simulink model "VCMGCM1962020b_v2"  (R2020b)
settings: Solver=FixedStepDiscrete  StartTime=0.0  StopTime=10.0  FixedStep=0.005  RelTol=1e-3  EnableMultiTasking=on
PreLoadFcn:
  | try, model_open; catch, disp('Error occurred while executing model pre-load callback: model_open.m'); disp('Please assure that the MATLAB working directory is set to the model directory before opening.'); end
InitFcn:
  | try, model_open; catch, end
undefined symbols (not defined in the file): Bridge, GCM, H, raptor_get_param_eval, raptor_get_safe_string, raptor_xcp_function
libraries: Blocks_lib x1165, Raptor_lib x665, simulink x62, VCM_lib x5
(part 6 of 23)

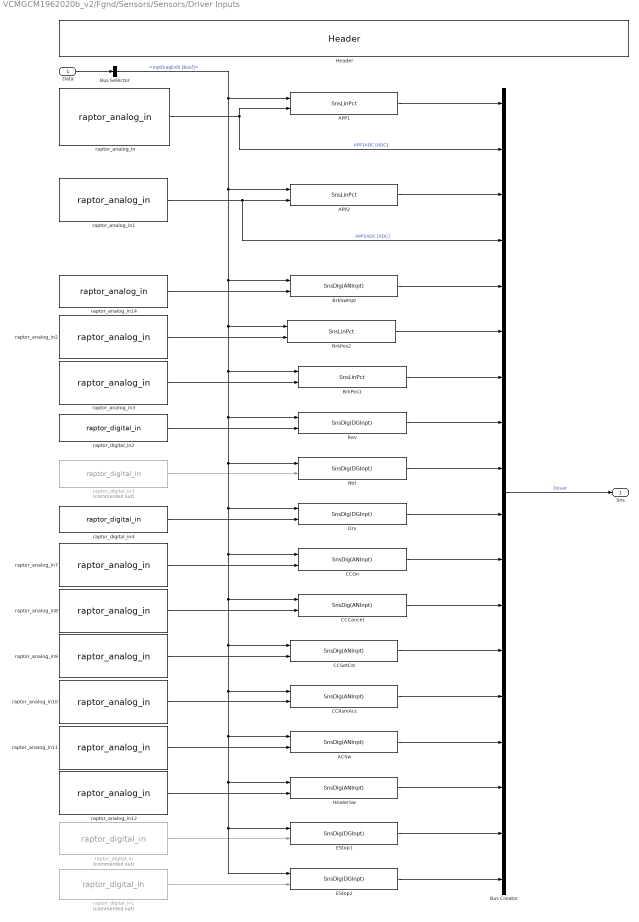
== system VCMGCM1962020b_v2/Fgnd/Sensors/Sensors/Driver Inputs ==
  Data : Inport
  ACSw : Blocks_lib/SnsDig(ANInpt)  nam='ACSw'  group='Sensors | Driver Input'  samptime=samptime
  APP1 : Blocks_lib/SnsLinPct  input=Analog  nam='APP1'  group='Sensors | Driver Input'  samptime=samptime
  APP2 : Blocks_lib/SnsLinPct  input=Analog  nam='APP2'  group='Sensors | Driver Input'  samptime=samptime
  BrkPos1 : Blocks_lib/SnsLinPct  input=Analog  nam='BrkPos1'  group='Sensors | Driver Input'  samptime=samptime
  BrkPos2 : Blocks_lib/SnsLinPct  input=Analog  nam='BrkPos2'  group='Sensors | Driver Input'  samptime=samptime
  BrkSwInpt : Blocks_lib/SnsDig(ANInpt)  nam='BrkSwInpt'  group='Sensors | Driver Input'  samptime=samptime
  Bus Creator : BusCreator  Inputs=18
  Bus Selector : BusSelector  OutputSignals=Control.Mode.StartStop.InptDiagEnbl [Bool]
  CCCancel : Blocks_lib/SnsDig(ANInpt)  nam='CCCancel'  group='Sensors | Driver Input'  samptime=samptime
  CCOn : Blocks_lib/SnsDig(ANInpt)  nam='CCOn'  group='Sensors | Driver Input'  samptime=samptime
  CCRsmAcc : Blocks_lib/SnsDig(ANInpt)  nam='CCRsmAcc'  group='Sensors | Driver Input'  samptime=samptime
  CCSetCst : Blocks_lib/SnsDig(ANInpt)  nam='CCSetCst'  group='Sensors | Driver Input'  samptime=samptime
  Drv : Blocks_lib/SnsDig(DGInpt)  nam='Drv'  group='Sensors | Driver Input'  samptime=samptime
  EStop1 : Blocks_lib/SnsDig(DGInpt)  nam='EStop1'  group='Sensors | Driver Input'  samptime=samptime
  EStop2 : Blocks_lib/SnsDig(DGInpt)  nam='EStop2'  group='Sensors | Driver Input'  samptime=samptime
  Header : Blocks_lib/Header  width=Portrait  addtext=''
  HeaterSw : Blocks_lib/SnsDig(ANInpt)  nam='HeaterSw'  group='Sensors | Driver Input'  samptime=samptime
  Ntrl : Blocks_lib/SnsDig(DGInpt)  nam='Ntrl'  group='Sensors | Driver Input'  samptime=samptime
  Rev : Blocks_lib/SnsDig(DGInpt)  nam='Rev'  group='Sensors | Driver Input'  samptime=samptime
  raptor_analog_in : Raptor_lib/Input & Output/raptor_analog_in  resourceValues=INPUT2|INPUT3|INPUT4|INPUT5|INPUT6|INPUT7|INPUT8|INPUT9|INPUT10|INPUT11|INPUT12|INPUT13|INPUT14|INPUT15|INPUT16|INPUT17|INPUT18|INPUT19|INPUT20|INPUT21|INPUT22|INPUT23|INPUT24|INPUT25|INPUT26|INPUT27|INPUT28|INPUT29|INPUT30|INPUT31|INPUT32|(None)  resource=INPUT30  pullUDValues=215k PD  pullUD=215k PD  rangeValues=0 - 5 V  range=0 - 5 V  filterrateValues=[]  filterrate='RAPTOR MASK DEFAULT'  resolutionValues=[]  resolution=[]
      settings: SourceProductName=Raptor
  raptor_analog_in1 : Raptor_lib/Input & Output/raptor_analog_in  resourceValues=INPUT2|INPUT3|INPUT4|INPUT5|INPUT6|INPUT7|INPUT8|INPUT9|INPUT10|INPUT11|INPUT12|INPUT13|INPUT14|INPUT15|INPUT16|INPUT17|INPUT18|INPUT19|INPUT20|INPUT21|INPUT22|INPUT23|INPUT24|INPUT25|INPUT26|INPUT27|INPUT28|INPUT29|INPUT30|INPUT31|INPUT32|(None)  resource=INPUT29  pullUDValues=215k PD  pullUD=215k PD  rangeValues=0 - 5 V  range=0 - 5 V  filterrateValues=[]  filterrate='RAPTOR MASK DEFAULT'  resolutionValues=[]  resolution=[]
      settings: SourceProductName=Raptor
  raptor_analog_in{7..10} (4 alike) : Raptor_lib/Input & Output/raptor_analog_in  resourceValues=INPUT2|INPUT3|INPUT4|INPUT5|INPUT6|INPUT7|INPUT8|INPUT9|INPUT10|INPUT11|INPUT12|INPUT13|INPUT14|INPUT15|INPUT16|INPUT17|INPUT18|INPUT19|INPUT20|INPUT21|INPUT22|INPUT23|INPUT24|INPUT25|INPUT26|INPUT27|INPUT28|INPUT29|INPUT30|INPUT31|INPUT32|(None)  resource=(None)  pullUDValues=(None)  pullUD=(None)  rangeValues=(None)  range=(None)  filterrateValues=[]  filterrate='RAPTOR MASK DEFAULT'  resolutionValues=[]  resolution=[]
      settings: SourceProductName=Raptor
  raptor_analog_in11 : Raptor_lib/Input & Output/raptor_analog_in  resourceValues=INPUT2|INPUT3|INPUT4|INPUT5|INPUT6|INPUT7|INPUT8|INPUT9|INPUT10|INPUT11|INPUT12|INPUT13|INPUT14|INPUT15|INPUT16|INPUT17|INPUT18|INPUT19|INPUT20|INPUT21|INPUT22|INPUT23|INPUT24|INPUT25|INPUT26|INPUT27|INPUT28|INPUT29|INPUT30|INPUT31|INPUT32|(None)  resource=INPUT8  pullUDValues=4.64k PU  pullUD=4.64k PU  rangeValues=0 - 5 V  range=0 - 5 V  filterrateValues=[]  filterrate='RAPTOR MASK DEFAULT'  resolutionValues=[]  resolution=[]
      settings: SourceProductName=Raptor
  raptor_analog_in12 : Raptor_lib/Input & Output/raptor_analog_in  resourceValues=INPUT2|INPUT3|INPUT4|INPUT5|INPUT6|INPUT7|INPUT8|INPUT9|INPUT10|INPUT11|INPUT12|INPUT13|INPUT14|INPUT15|INPUT16|INPUT17|INPUT18|INPUT19|INPUT20|INPUT21|INPUT22|INPUT23|INPUT24|INPUT25|INPUT26|INPUT27|INPUT28|INPUT29|INPUT30|INPUT31|INPUT32|(None)  resource=INPUT16  pullUDValues=4.64k PU  pullUD=4.64k PU  rangeValues=0 - 5 V  range=0 - 5 V  filterrateValues=[]  filterrate='RAPTOR MASK DEFAULT'  resolutionValues=[]  resolution=[]
      settings: SourceProductName=Raptor
  raptor_analog_in14 : Raptor_lib/Input & Output/raptor_analog_in  resourceValues=INPUT2|INPUT3|INPUT4|INPUT5|INPUT6|INPUT7|INPUT8|INPUT9|INPUT10|INPUT11|INPUT12|INPUT13|INPUT14|INPUT15|INPUT16|INPUT17|INPUT18|INPUT19|INPUT20|INPUT21|INPUT22|INPUT23|INPUT24|INPUT25|INPUT26|INPUT27|INPUT28|INPUT29|INPUT30|INPUT31|INPUT32|(None)  resource=INPUT17  pullUDValues=422k PD  pullUD=422k PD  rangeValues=0 - 5 V  range=0 - 5 V  filterrateValues=[]  filterrate='RAPTOR MASK DEFAULT'  resolutionValues=[]  resolution=[]
      settings: SourceProductName=Raptor
  raptor_analog_in2 : Raptor_lib/Input & Output/raptor_analog_in  resourceValues=INPUT2|INPUT3|INPUT4|INPUT5|INPUT6|INPUT7|INPUT8|INPUT9|INPUT10|INPUT11|INPUT12|INPUT13|INPUT14|INPUT15|INPUT16|INPUT17|INPUT18|INPUT19|INPUT20|INPUT21|INPUT22|INPUT23|INPUT24|INPUT25|INPUT26|INPUT27|INPUT28|INPUT29|INPUT30|INPUT31|INPUT32|(None)  resource=INPUT24  pullUDValues=56.7k PD  pullUD=56.7k PD  rangeValues=0 - 5 V  range=0 - 5 V  filterrateValues=[]  filterrate='RAPTOR MASK DEFAULT'  resolutionValues=[]  resolution=[]
      settings: SourceProductName=Raptor
  raptor_analog_in3 : Raptor_lib/Input & Output/raptor_analog_in  resourceValues=INPUT2|INPUT3|INPUT4|INPUT5|INPUT6|INPUT7|INPUT8|INPUT9|INPUT10|INPUT11|INPUT12|INPUT13|INPUT14|INPUT15|INPUT16|INPUT17|INPUT18|INPUT19|INPUT20|INPUT21|INPUT22|INPUT23|INPUT24|INPUT25|INPUT26|INPUT27|INPUT28|INPUT29|INPUT30|INPUT31|INPUT32|(None)  resource=INPUT23  pullUDValues=56.7k PD  pullUD=56.7k PD  rangeValues=0 - 5 V  range=0 - 5 V  filterrateValues=[]  filterrate='RAPTOR MASK DEFAULT'  resolutionValues=[]  resolution=[]
      settings: SourceProductName=Raptor
  raptor_digital_in : Raptor_lib/Input & Output/raptor_digital_in  Commented=on  resourceValues=WAKE_INPUT1|INPUT33|INPUT34|INPUT35|INPUT36|INPUT37|INPUT38|INPUT39|INPUT40|(None)  resource=INPUT37  pullUDValues=1.3k PU  pullUD=1.3k PU  upperThres='RAPTOR MASK DEFAULT'  lowerThres='RAPTOR MASK DEFAULT'
      settings: SourceProductName=Raptor
  raptor_digital_in1 : Raptor_lib/Input & Output/raptor_digital_in  Commented=on  resourceValues=WAKE_INPUT1|INPUT33|INPUT34|INPUT35|INPUT36|INPUT37|INPUT38|INPUT39|INPUT40|(None)  resource=INPUT39  pullUDValues=1.3k PU  pullUD=1.3k PU  upperThres='RAPTOR MASK DEFAULT'  lowerThres='RAPTOR MASK DEFAULT'
      settings: SourceProductName=Raptor
  raptor_digital_in2 : Raptor_lib/Input & Output/raptor_digital_in  resourceValues=WAKE_INPUT1|INPUT33|INPUT34|INPUT35|INPUT36|INPUT37|INPUT38|INPUT39|INPUT40|(None)  resource=INPUT34  pullUDValues=1.3k PD  pullUD=1.3k PD  upperThres='RAPTOR MASK DEFAULT'  lowerThres='RAPTOR MASK DEFAULT'
      settings: SourceProductName=Raptor
  raptor_digital_in3 : Raptor_lib/Input & Output/raptor_digital_in  Commented=on  resourceValues=WAKE_INPUT1|INPUT33|INPUT34|INPUT35|INPUT36|INPUT37|INPUT38|INPUT39|INPUT40|(None)  resource=INPUT33  pullUDValues=1.3k PD  pullUD=1.3k PD  upperThres='RAPTOR MASK DEFAULT'  lowerThres='RAPTOR MASK DEFAULT'
      settings: SourceProductName=Raptor
  raptor_digital_in4 : Raptor_lib/Input & Output/raptor_digital_in  resourceValues=WAKE_INPUT1|INPUT33|INPUT34|INPUT35|INPUT36|INPUT37|INPUT38|INPUT39|INPUT40|(None)  resource=INPUT35  pullUDValues=1.3k PD  pullUD=1.3k PD  upperThres='RAPTOR MASK DEFAULT'  lowerThres='RAPTOR MASK DEFAULT'
      settings: SourceProductName=Raptor
  Sns : Outport  VectorParamsAs1DForOutWhenUnconnected=off
  wires:
  raptor_analog_in12/1 -> HeaterSw/2
  raptor_analog_in11/1 -> ACSw/2
  HeaterSw/1 -> Bus Creator/16
  ACSw/1 -> Bus Creator/15
  raptor_digital_in/1 -> EStop1/2
  EStop1/1 -> Bus Creator/17
  raptor_digital_in1/1 -> EStop2/2
  EStop2/1 -> Bus Creator/18
  CCRsmAcc/1 -> Bus Creator/14
  CCSetCst/1 -> Bus Creator/13
  CCCancel/1 -> Bus Creator/12
  CCOn/1 -> Bus Creator/11
  Drv/1 -> Bus Creator/10
  Ntrl/1 -> Bus Creator/9
  Rev/1 -> Bus Creator/8
  BrkPos1/1 -> Bus Creator/7
  APP2/1 -> Bus Creator/3
  raptor_analog_in1/1 -> Bus Creator/4, APP2/2  "APP2ADC [ADC]"
  raptor_analog_in/1 -> APP1/2, Bus Creator/2  "APP1ADC [ADC]"
  raptor_analog_in9/1 -> CCSetCst/2
  raptor_analog_in10/1 -> CCRsmAcc/2
  raptor_analog_in8/1 -> CCCancel/2
  raptor_analog_in7/1 -> CCOn/2
  raptor_digital_in4/1 -> Drv/2
  raptor_digital_in3/1 -> Ntrl/2
  raptor_digital_in2/1 -> Rev/2
  raptor_analog_in2/1 -> BrkPos2/2
  Bus Creator/1 -> Sns/1  "Driver"
  APP1/1 -> Bus Creator/1
  Data/1 -> Bus Selector/1
  Bus Selector/1 -> EStop2/1, EStop1/1, HeaterSw/1, ACSw/1, CCRsmAcc/1, CCSetCst/1, CCCancel/1, CCOn/1, Drv/1, Ntrl/1, Rev/1, BrkPos1/1, BrkPos2/1, BrkSwInpt/1, APP2/1, APP1/1  "<InptDiagEnbl [Bool]>"
  BrkPos2/1 -> Bus Creator/6
  raptor_analog_in14/1 -> BrkSwInpt/2
  BrkSwInpt/1 -> Bus Creator/5
  raptor_analog_in3/1 -> BrkPos1/2

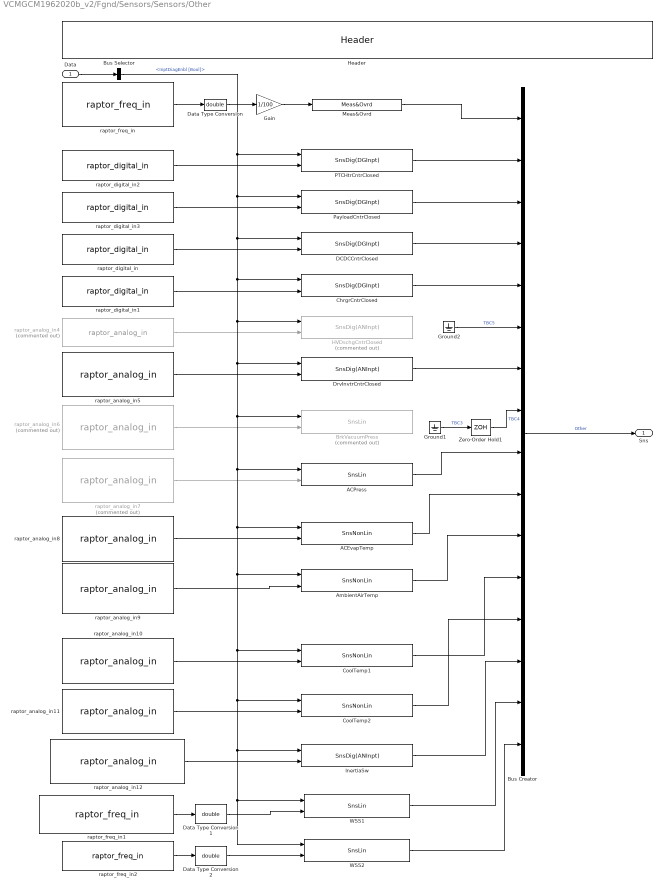
== system VCMGCM1962020b_v2/Fgnd/Sensors/Sensors/Other ==
  Data : Inport
  ACEvapTemp : Blocks_lib/SnsNonLin  input=Analog  nam='ACEvapTemp'  units='degC'  len=11  group='Sensors | Other'  samptime=samptime
  ACPress : Blocks_lib/SnsLin  input=Analog  nam='ACPress'  units='kPa'  group='Sensors | Other'  samptime=samptime
  AmbientAirTemp : Blocks_lib/SnsNonLin  input=Analog  nam='AmbientAirTemp'  units='degC'  len=8  group='Sensors | Other'  samptime=samptime
  BrkVacuumPress : Blocks_lib/SnsLin  Commented=on  input=Analog  nam='BrkVacuumPress'  units='kPa'  group='Sensors | Other'  samptime=samptime
  Bus Creator : BusCreator  Inputs=16
  Bus Selector : BusSelector  OutputSignals=Control.Mode.StartStop.InptDiagEnbl [Bool]
  ChrgrCntrClosed : Blocks_lib/SnsDig(DGInpt)  nam='ChrgrCntrClosed'  group='Sensors | Driver Input'  samptime=samptime
  CoolTemp1 : Blocks_lib/SnsNonLin  input=Analog  nam='CoolTemp1'  units='degC'  len=11  group='Sensors | Other'  samptime=samptime
  CoolTemp2 : Blocks_lib/SnsNonLin  input=Analog  nam='CoolTemp2'  units='degC'  len=11  group='Sensors | Other'  samptime=samptime
  DCDCCntrClosed : Blocks_lib/SnsDig(DGInpt)  nam='DCDCCntrClosed'  group='Sensors | Driver Input'  samptime=samptime
  Data Type Conversion : DataTypeConversion  OutDataTypeStr=double
  Data Type Conversion1 : DataTypeConversion  OutDataTypeStr=double
  Data Type Conversion2 : DataTypeConversion  OutDataTypeStr=double
  DrvInvtrCntrClosed : Blocks_lib/SnsDig(ANInpt)  nam='DrvInvtrCntrClosed'  group='Sensors | Other'  samptime=samptime
  Gain : Gain  Gain=1/100
  Ground1 : Ground
  Ground2 : Ground
  HVDschgCntrClosed : Blocks_lib/SnsDig(ANInpt)  Commented=on  nam='HVDschgCntrClosed'  group='Sensors | Other'  samptime=samptime
  Header : Blocks_lib/Header  width=Portrait  addtext=''
  InertiaSw : Blocks_lib/SnsDig(ANInpt)  nam='InertiaSw'  group='Sensors | Other'  samptime=samptime
  Meas&Ovrd : Blocks_lib/Meas&Ovrd  nam='HVILInFrq'  name_source=Parameter  view_as=Number  enum_struct={}  gain=1  min=-inf  max=inf  precision=''  units='Hz'  help='HVIL in frequency'  group='Sensors | Other'
  PTCHtrCntrClosed : Blocks_lib/SnsDig(DGInpt)  nam='PTCHtrCntrClosed'  group='Sensors | Driver Input'  samptime=samptime
  PayloadCntrClosed : Blocks_lib/SnsDig(DGInpt)  nam='PayloadCntrClosed'  group='Sensors | Driver Input'  samptime=samptime
  WSS1 : Blocks_lib/SnsLin  input=Analog  nam='WSS1'  units='RPM'  group='Sensors | Other'  samptime=samptime
  WSS2 : Blocks_lib/SnsLin  input=Analog  nam='WSS2'  units='RPM'  group='Sensors | Other'  samptime=samptime
  Zero-Order Hold1 : ZeroOrderHold  SampleTime=-1
  raptor_analog_in10 : Raptor_lib/Input & Output/raptor_analog_in  resourceValues=INPUT2|INPUT3|INPUT4|INPUT5|INPUT6|INPUT7|INPUT8|INPUT9|INPUT10|INPUT11|INPUT12|INPUT13|INPUT14|INPUT15|INPUT16|INPUT17|INPUT18|INPUT19|INPUT20|INPUT21|INPUT22|INPUT23|INPUT24|INPUT25|INPUT26|INPUT27|INPUT28|INPUT29|INPUT30|INPUT31|INPUT32|(None)  resource=INPUT21  pullUDValues=2.15k PU  pullUD=2.15k PU  rangeValues=0 - 5 V  range=0 - 5 V  filterrateValues=[]  filterrate='RAPTOR MASK DEFAULT'  resolutionValues=[]  resolution=[]
      settings: SourceProductName=Raptor
  raptor_analog_in11 : Raptor_lib/Input & Output/raptor_analog_in  resourceValues=INPUT2|INPUT3|INPUT4|INPUT5|INPUT6|INPUT7|INPUT8|INPUT9|INPUT10|INPUT11|INPUT12|INPUT13|INPUT14|INPUT15|INPUT16|INPUT17|INPUT18|INPUT19|INPUT20|INPUT21|INPUT22|INPUT23|INPUT24|INPUT25|INPUT26|INPUT27|INPUT28|INPUT29|INPUT30|INPUT31|INPUT32|(None)  resource=INPUT22  pullUDValues=2.15k PU  pullUD=2.15k PU  rangeValues=0 - 5 V  range=0 - 5 V  filterrateValues=[]  filterrate='RAPTOR MASK DEFAULT'  resolutionValues=[]  resolution=[]
      settings: SourceProductName=Raptor
  raptor_analog_in12 : Raptor_lib/Input & Output/raptor_analog_in  resourceValues=INPUT2|INPUT3|INPUT4|INPUT5|INPUT6|INPUT7|INPUT8|INPUT9|INPUT10|INPUT11|INPUT12|INPUT13|INPUT14|INPUT15|INPUT16|INPUT17|INPUT18|INPUT19|INPUT20|INPUT21|INPUT22|INPUT23|INPUT24|INPUT25|INPUT26|INPUT27|INPUT28|INPUT29|INPUT30|INPUT31|INPUT32|(None)  resource=INPUT19  pullUDValues=2.15k PU  pullUD=2.15k PU  rangeValues=0 - 5 V  range=0 - 5 V  filterrateValues=[]  filterrate='RAPTOR MASK DEFAULT'  resolutionValues=[]  resolution=[]
      settings: SourceProductName=Raptor
  raptor_analog_in4 : Raptor_lib/Input & Output/raptor_analog_in  Commented=on  resourceValues=INPUT2|INPUT3|INPUT4|INPUT5|INPUT6|INPUT7|INPUT8|INPUT9|INPUT10|INPUT11|INPUT12|INPUT13|INPUT14|INPUT15|INPUT16|INPUT17|INPUT18|INPUT19|INPUT20|INPUT21|INPUT22|INPUT23|INPUT24|INPUT25|INPUT26|INPUT27|INPUT28|INPUT29|INPUT30|INPUT31|INPUT32|(None)  resource=INPUT10  pullUDValues=681k PU  pullUD=681k PU  rangeValues=0 - 5 V  range=0 - 5 V  filterrateValues=[]  filterrate='RAPTOR MASK DEFAULT'  resolutionValues=[]  resolution=[]
      settings: SourceProductName=Raptor
  raptor_analog_in5 : Raptor_lib/Input & Output/raptor_analog_in  resourceValues=INPUT2|INPUT3|INPUT4|INPUT5|INPUT6|INPUT7|INPUT8|INPUT9|INPUT10|INPUT11|INPUT12|INPUT13|INPUT14|INPUT15|INPUT16|INPUT17|INPUT18|INPUT19|INPUT20|INPUT21|INPUT22|INPUT23|INPUT24|INPUT25|INPUT26|INPUT27|INPUT28|INPUT29|INPUT30|INPUT31|INPUT32|(None)  resource=INPUT11  pullUDValues=681k PU  pullUD=681k PU  rangeValues=0 - 5 V  range=0 - 5 V  filterrateValues=[]  filterrate='RAPTOR MASK DEFAULT'  resolutionValues=[]  resolution=[]
      settings: SourceProductName=Raptor
  raptor_analog_in6 : Raptor_lib/Input & Output/raptor_analog_in  Commented=on  resourceValues=INPUT2|INPUT3|INPUT4|INPUT5|INPUT6|INPUT7|INPUT8|INPUT9|INPUT10|INPUT11|INPUT12|INPUT13|INPUT14|INPUT15|INPUT16|INPUT17|INPUT18|INPUT19|INPUT20|INPUT21|INPUT22|INPUT23|INPUT24|INPUT25|INPUT26|INPUT27|INPUT28|INPUT29|INPUT30|INPUT31|INPUT32|(None)  resource=INPUT23  pullUDValues=56.7k PD  pullUD=56.7k PD  rangeValues=0 - 5 V  range=0 - 5 V  filterrateValues=[]  filterrate='RAPTOR MASK DEFAULT'  resolutionValues=[]  resolution=[]
      settings: SourceProductName=Raptor
  raptor_analog_in7 : Raptor_lib/Input & Output/raptor_analog_in  Commented=on  resourceValues=INPUT2|INPUT3|INPUT4|INPUT5|INPUT6|INPUT7|INPUT8|INPUT9|INPUT10|INPUT11|INPUT12|INPUT13|INPUT14|INPUT15|INPUT16|INPUT17|INPUT18|INPUT19|INPUT20|INPUT21|INPUT22|INPUT23|INPUT24|INPUT25|INPUT26|INPUT27|INPUT28|INPUT29|INPUT30|INPUT31|INPUT32|(None)  resource=INPUT24  pullUDValues=56.7k PD  pullUD=56.7k PD  rangeValues=0 - 5 V  range=0 - 5 V  filterrateValues=[]  filterrate='RAPTOR MASK DEFAULT'  resolutionValues=[]  resolution=[]
      settings: SourceProductName=Raptor
  raptor_analog_in8 : Raptor_lib/Input & Output/raptor_analog_in  resourceValues=INPUT2|INPUT3|INPUT4|INPUT5|INPUT6|INPUT7|INPUT8|INPUT9|INPUT10|INPUT11|INPUT12|INPUT13|INPUT14|INPUT15|INPUT16|INPUT17|INPUT18|INPUT19|INPUT20|INPUT21|INPUT22|INPUT23|INPUT24|INPUT25|INPUT26|INPUT27|INPUT28|INPUT29|INPUT30|INPUT31|INPUT32|(None)  resource=INPUT27  pullUDValues=2.15k PU  pullUD=2.15k PU  rangeValues=0 - 5 V  range=0 - 5 V  filterrateValues=[]  filterrate='RAPTOR MASK DEFAULT'  resolutionValues=[]  resolution=[]
      settings: SourceProductName=Raptor
  raptor_analog_in9 : Raptor_lib/Input & Output/raptor_analog_in  resourceValues=INPUT2|INPUT3|INPUT4|INPUT5|INPUT6|INPUT7|INPUT8|INPUT9|INPUT10|INPUT11|INPUT12|INPUT13|INPUT14|INPUT15|INPUT16|INPUT17|INPUT18|INPUT19|INPUT20|INPUT21|INPUT22|INPUT23|INPUT24|INPUT25|INPUT26|INPUT27|INPUT28|INPUT29|INPUT30|INPUT31|INPUT32|(None)  resource=INPUT28  pullUDValues=2.15k PU  pullUD=2.15k PU  rangeValues=0 - 5 V  range=0 - 5 V  filterrateValues=[]  filterrate='RAPTOR MASK DEFAULT'  resolutionValues=[]  resolution=[]
      settings: SourceProductName=Raptor
  raptor_digital_in : Raptor_lib/Input & Output/raptor_digital_in  resourceValues=WAKE_INPUT1|INPUT33|INPUT34|INPUT35|INPUT36|INPUT37|INPUT38|INPUT39|INPUT40|(None)  resource=INPUT37  pullUDValues=1.3k PU  pullUD=1.3k PU  upperThres='RAPTOR MASK DEFAULT'  lowerThres='RAPTOR MASK DEFAULT'
      settings: SourceProductName=Raptor
  raptor_digital_in1 : Raptor_lib/Input & Output/raptor_digital_in  resourceValues=WAKE_INPUT1|INPUT33|INPUT34|INPUT35|INPUT36|INPUT37|INPUT38|INPUT39|INPUT40|(None)  resource=INPUT38  pullUDValues=1.18k PU  pullUD=1.18k PU  upperThres='RAPTOR MASK DEFAULT'  lowerThres='RAPTOR MASK DEFAULT'
      settings: SourceProductName=Raptor
  raptor_digital_in2 : Raptor_lib/Input & Output/raptor_digital_in  resourceValues=WAKE_INPUT1|INPUT33|INPUT34|INPUT35|INPUT36|INPUT37|INPUT38|INPUT39|INPUT40|(None)  resource=INPUT39  pullUDValues=1.3k PU  pullUD=1.3k PU  upperThres='RAPTOR MASK DEFAULT'  lowerThres='RAPTOR MASK DEFAULT'
      settings: SourceProductName=Raptor
  raptor_digital_in3 : Raptor_lib/Input & Output/raptor_digital_in  resourceValues=WAKE_INPUT1|INPUT33|INPUT34|INPUT35|INPUT36|INPUT37|INPUT38|INPUT39|INPUT40|(None)  resource=INPUT40  pullUDValues=1.3k PU  pullUD=1.3k PU  upperThres='RAPTOR MASK DEFAULT'  lowerThres='RAPTOR MASK DEFAULT'
      settings: SourceProductName=Raptor
  raptor_freq_in : Raptor_lib/Input & Output/raptor_freq_in  resourceValues=(None)|INPUT41|INPUT42|INPUT43|INPUT44|INPUT45  resource=INPUT41  hasDuty=off  pullUDValues=[]  pullUD=[]  interfaceValues=[]  interface=[]  hasEdgeCount='RAPTOR MASK DEFAULT'
      settings: SourceProductName=Raptor
  raptor_freq_in1 : Raptor_lib/Input & Output/raptor_freq_in  resourceValues=INPUT41|INPUT42|INPUT43|INPUT44|INPUT45|(None)  resource=INPUT42  hasDuty=off  pullUDValues=[]  pullUD=[]  interfaceValues=[]  interface=[]  hasEdgeCount='RAPTOR MASK DEFAULT'
      settings: SourceProductName=Raptor
  raptor_freq_in2 : Raptor_lib/Input & Output/raptor_freq_in  resourceValues=INPUT41|INPUT42|INPUT43|INPUT44|INPUT45|(None)  resource=INPUT45  hasDuty=off  pullUDValues=[]  pullUD=[]  interfaceValues=[]  interface=[]  hasEdgeCount='RAPTOR MASK DEFAULT'
      settings: SourceProductName=Raptor
  Sns : Outport  VectorParamsAs1DForOutWhenUnconnected=off
  wires:
  raptor_analog_in10/1 -> CoolTemp1/2
  raptor_digital_in3/1 -> PayloadCntrClosed/2
  raptor_digital_in2/1 -> PTCHtrCntrClosed/2
  raptor_analog_in5/1 -> DrvInvtrCntrClosed/2
  raptor_digital_in/1 -> DCDCCntrClosed/2
  raptor_analog_in4/1 -> HVDschgCntrClosed/2
  raptor_digital_in1/1 -> ChrgrCntrClosed/2
  raptor_analog_in9/1 -> AmbientAirTemp/2
  raptor_analog_in8/1 -> ACEvapTemp/2
  raptor_analog_in7/1 -> ACPress/2
  raptor_analog_in11/1 -> CoolTemp2/2
  raptor_analog_in6/1 -> BrkVacuumPress/2
  Bus Creator/1 -> Sns/1  "Other"
  Bus Selector/1 -> PTCHtrCntrClosed/1, CoolTemp1/1, CoolTemp2/1, WSS2/1, WSS1/1, InertiaSw/1, AmbientAirTemp/1, ACEvapTemp/1, ACPress/1, BrkVacuumPress/1, DrvInvtrCntrClosed/1, HVDschgCntrClosed/1, ChrgrCntrClosed/1, DCDCCntrClosed/1, PayloadCntrClosed/1  "<InptDiagEnbl [Bool]>"
  Data/1 -> Bus Selector/1
  Gain/1 -> Meas&Ovrd/1
  Data Type Conversion/1 -> Gain/1
  raptor_freq_in/1 -> Data Type Conversion/1
  Meas&Ovrd/1 -> Bus Creator/1
  DCDCCntrClosed/1 -> Bus Creator/4
  ChrgrCntrClosed/1 -> Bus Creator/5
  ACPress/1 -> Bus Creator/9
  ACEvapTemp/1 -> Bus Creator/10
  AmbientAirTemp/1 -> Bus Creator/11
  CoolTemp1/1 -> Bus Creator/12
  InertiaSw/1 -> Bus Creator/14
  raptor_analog_in12/1 -> InertiaSw/2
  CoolTemp2/1 -> Bus Creator/13
  Ground1/1 -> Zero-Order Hold1/1  "TBC3"
  Zero-Order Hold1/1 -> Bus Creator/8  "TBC4"
  Ground2/1 -> Bus Creator/6  "TBC5"
  PTCHtrCntrClosed/1 -> Bus Creator/2
  PayloadCntrClosed/1 -> Bus Creator/3
  DrvInvtrCntrClosed/1 -> Bus Creator/7
  raptor_freq_in2/1 -> Data Type Conversion2/1
  raptor_freq_in1/1 -> Data Type Conversion1/1
  Data Type Conversion1/1 -> WSS1/2
  Data Type Conversion2/1 -> WSS2/2
  WSS1/1 -> Bus Creator/15
  WSS2/1 -> Bus Creator/16

== system VCMGCM1962020b_v2/Fgnd/Sensors/Sensors/Voltage ==
  Data : Inport
  Bus Creator : BusCreator  Inputs=4
  Bus Selector : BusSelector  OutputSignals=Control.Mode.StartStop.InptDiagEnbl [Bool]
  DRVPVolt : Blocks_lib/SnsLin(w//oDiag)  input=Analog  nam='DRVPVolt'  units='V'  group='Sensors | Voltage'  samptime=samptime
  Header : Blocks_lib/Header  width=Portrait  addtext=''
  WakeChgr : Blocks_lib/SnsDig(DGInpt)  nam='WakeChgr'  group='Sensors | Voltage'  samptime=samptime
  XDRPVolt : Blocks_lib/SnsLin  input=Analog  nam='XDRPVolt'  units='V'  group='Sensors | Voltage'  samptime=samptime
  raptor_data_read : Raptor_lib/Data Storage/raptor_data_read  dataName='Wake_Bgnd'  dataShape=Scalar  idxSource=Input  idxRow=1  idxCol=1
      settings: SourceProductName=Raptor
  raptor_digital_in : Raptor_lib/Input & Output/raptor_digital_in  resourceValues=WAKE_INPUT1|INPUT33|INPUT34|INPUT35|INPUT36|INPUT37|INPUT38|INPUT39|INPUT40|(None)  resource=INPUT33  pullUDValues=1.3k PD  pullUD=1.3k PD  upperThres='RAPTOR MASK DEFAULT'  lowerThres='RAPTOR MASK DEFAULT'
      settings: SourceProductName=Raptor
  raptor_internal_measurement : Raptor_lib/Input & Output/raptor_internal_measurement  resourceValues=(None)|BATTERY_VOLTAGE  resource=BATTERY_VOLTAGE  out_eng=0  soft_filter=1  out_bool=0
      settings: SourceProductName=Raptor
  raptor_internal_measurement1 : Raptor_lib/Input & Output/raptor_internal_measurement  resourceValues=BATTERY_VOLTAGE|VSENS_SUPPLY|(None)  resource=VSENS_SUPPLY  out_eng=0  soft_filter=1  out_bool=0
      settings: SourceProductName=Raptor
  Sns : Outport  VectorParamsAs1DForOutWhenUnconnected=off
  wires:
  raptor_digital_in/1 -> WakeChgr/2
  WakeChgr/1 -> Bus Creator/2
  raptor_internal_measurement1/1 -> XDRPVolt/2
  raptor_internal_measurement/1 -> DRVPVolt/2
  Bus Creator/1 -> Sns/1  "Volt"
  XDRPVolt/1 -> Bus Creator/4
  DRVPVolt/1 -> Bus Creator/3
  raptor_data_read/1 -> Bus Creator/1  "Wake [Bool]"
  Data/1 -> Bus Selector/1
  Bus Selector/1 -> WakeChgr/1, DRVPVolt/1, XDRPVolt/1  "<InptDiagEnbl [Bool]>"

== system VCMGCM1962020b_v2/Fgnd/Virtual Sensors/Battery/Average ==
  Min : Inport
  Max : Inport  Port=2
  Add : Sum
  Constant : Constant  Value=2
  Divide : Product  Inputs=*/
  Avg : Outport
  wires:
  Min/1 -> Add/1
  Max/1 -> Add/2
  Add/1 -> Divide/1
  Constant/1 -> Divide/2
  Divide/1 -> Avg/1

== system VCMGCM1962020b_v2/Fgnd/Virtual Sensors/Battery/BattCCL ==
  Data : Inport
  Bus Selector : BusSelector  OutputSignals=Sensors.CAN.Batt.BMS1_Currents.Batt_CrntCHG_Cont.Batt_CrntCHG_ContVld [Bool],Sensors.CAN.Batt.BMS1_Currents.Batt_CrntCHG_Cont.Batt_CrntCHG_Cont []
  Header : Blocks_lib/Header  width=Portrait  addtext=''
  MinMax : MinMax  Inputs=2
  Product : Product
  Zero-Order Hold : ZeroOrderHold  SampleTime=-1
  raptor_adjustment : Raptor_lib/Data Storage/raptor_adjustment  paramName='BattCCLMultp'  nameSource=Parameter  initValue=0  dataType=double  storage=Calibration  calDispType=Number  calEnum={'Disabled', 'Enabled'}  calGain=1  calOffset=0  calMax=inf  calMin=-inf  calFormat=''  calUnit='multp'  calHelp='Battery charge current limit multiplier'  calAccess=1  calFunction='Virtual Sensors | Battery'  calDispHeaders=off  calColHeaders={'Col1' 'Col2' 'Col3'}  calRowHeaders={'Row1' 'Row2' 'Row3'}
      settings: SourceProductName=Raptor
  raptor_adjustment1 : Raptor_lib/Data Storage/raptor_adjustment  paramName='BattCCL_cal'  nameSource=Parameter  initValue=0  dataType=double  storage=Calibration  calDispType=Number  calEnum={'Disabled', 'Enabled'}  calGain=1  calOffset=0  calMax=inf  calMin=-inf  calFormat=''  calUnit='A'  calHelp='Battery charge current limit'  calAccess=1  calFunction='Virtual Sensors | Battery'  calDispHeaders=off  calColHeaders={'Col1' 'Col2' 'Col3'}  calRowHeaders={'Row1' 'Row2' 'Row3'}
      settings: SourceProductName=Raptor
  raptor_measurement : Raptor_lib/Data Storage/raptor_measurement  paramName='BattCCLFinal'  nameSource=Parameter  calDispType=Number  calEnum={'Disabled', 'Enabled'}  calGain=1  calOffset=0  calMax=inf  calMin=-inf  calFormat=''  calUnit='A'  calHelp='Battery charge current limit'  calAccess=1  calFunction='Virtual Sensors | Battery'  calVisible=on
      settings: SourceProductName=Raptor
  Vld : Outport  VectorParamsAs1DForOutWhenUnconnected=off
  A : Outport  Port=2  VectorParamsAs1DForOutWhenUnconnected=off
  wires:
  Bus Selector/2 -> Product/1  "<Batt_CrntCHG_Cont []>"
  Data/1 -> Bus Selector/1
  Zero-Order Hold/1 -> Vld/1
  Bus Selector/1 -> Zero-Order Hold/1  "<Batt_CrntCHG_ContVld [Bool]>"
  MinMax/1 -> A/1, raptor_measurement/1
  raptor_adjustment/1 -> Product/2
  raptor_adjustment1/1 -> MinMax/2
  Product/1 -> MinMax/1

== system VCMGCM1962020b_v2/Fgnd/Virtual Sensors/Battery/BattChgComplete ==
  Data : Inport
  Bus Selector : BusSelector  OutputSignals=Sensors.CAN.Batt.HVES1_Data2.Batt_SOC.Batt_SOCVld [Bool],Sensors.CAN.Batt.HVES1_Data2.Batt_SOC.Batt_SOC [%]
  Header : Blocks_lib/Header  width=Portrait  addtext=''
  Logical Operator : Logic  OutDataTypeStr=boolean
  Relational Operator : RelationalOperator  OutDataTypeStr=boolean  RndMeth=Simplest
  raptor_adjustment : Raptor_lib/Data Storage/raptor_adjustment  paramName='BattSOCLimt'  nameSource=Parameter  initValue=0  dataType=double  storage=Calibration  calDispType=Number  calEnum={'BMS', 'Model'}  calGain=1  calOffset=0  calMax=inf  calMin=-inf  calFormat=''  calUnit='%'  calHelp='Battery SOC to terminate Charging'  calAccess=1  calFunction='Virtual Sensors | Battery'  calDispHeaders=off  calColHeaders={'Col1' 'Col2' 'Col3'}  calRowHeaders={'Row1' 'Row2' 'Row3'}
      settings: SourceProductName=Raptor
  Bool : Outport  VectorParamsAs1DForOutWhenUnconnected=off
  wires:
  Logical Operator/1 -> Bool/1
  Bus Selector/1 -> Logical Operator/1  "<Batt_SOCVld [Bool]>"
  Data/1 -> Bus Selector/1
  Relational Operator/1 -> Logical Operator/2
  Bus Selector/2 -> Relational Operator/1  "<Batt_SOC [%]>"
  raptor_adjustment/1 -> Relational Operator/2

== system VCMGCM1962020b_v2/Fgnd/Virtual Sensors/Battery/BattDCL ==
  note: Space to add continous
      | current limit from batterypack
  CrntLmtVld : Inport
  CrntLmt : Inport  Port=2
  Header : Blocks_lib/Header  width=Portrait  addtext=''
  MinMax : MinMax  Inputs=2
  Zero-Order Hold : ZeroOrderHold  SampleTime=-1
  raptor_adjustment1 : Raptor_lib/Data Storage/raptor_adjustment  paramName='BattDCL_cal'  nameSource=Parameter  initValue=0  dataType=double  storage=Calibration  calDispType=Number  calEnum={'Disabled', 'Enabled'}  calGain=1  calOffset=0  calMax=inf  calMin=-inf  calFormat=''  calUnit='A'  calHelp='Battery discharge current limit'  calAccess=1  calFunction='Virtual Sensors | Battery'  calDispHeaders=off  calColHeaders={'Col1' 'Col2' 'Col3'}  calRowHeaders={'Row1' 'Row2' 'Row3'}
      settings: SourceProductName=Raptor
  raptor_measurement : Raptor_lib/Data Storage/raptor_measurement  paramName='BattDCLFinal'  nameSource=Parameter  calDispType=Number  calEnum={'Disabled', 'Enabled'}  calGain=1  calOffset=0  calMax=inf  calMin=-inf  calFormat=''  calUnit='A'  calHelp='Battery discharge current limit'  calAccess=1  calFunction='Virtual Sensors | Battery'  calVisible=on
      settings: SourceProductName=Raptor
  Vld : Outport  VectorParamsAs1DForOutWhenUnconnected=off
  A : Outport  Port=2  VectorParamsAs1DForOutWhenUnconnected=off
  wires:
  MinMax/1 -> raptor_measurement/1, A/1
  CrntLmtVld/1 -> Zero-Order Hold/1
  Zero-Order Hold/1 -> Vld/1
  raptor_adjustment1/1 -> MinMax/2
  CrntLmt/1 -> MinMax/1

== system VCMGCM1962020b_v2/Fgnd/Virtual Sensors/Battery/BattFault ==
  Data : Inport
  Bus Selector : BusSelector  OutputSignals=Sensors.CAN.Batt.BMS4_MasterStatus.Batt_Fault.Batt_FaultVld [Bool],Sensors.CAN.Batt.BMS4_MasterStatus.Batt_Fault.Batt_Fault []
  Header : Blocks_lib/Header  width=Portrait  addtext=''
  Zero-Order Hold : ZeroOrderHold  SampleTime=-1
  Vld : Outport  VectorParamsAs1DForOutWhenUnconnected=off
  Bool : Outport  Port=2  VectorParamsAs1DForOutWhenUnconnected=off
  wires:
  Data/1 -> Bus Selector/1
  Bus Selector/2 -> Bool/1  "<Batt_Fault []>"
  Zero-Order Hold/1 -> Vld/1
  Bus Selector/1 -> Zero-Order Hold/1  "<Batt_FaultVld [Bool]>"

== system VCMGCM1962020b_v2/Fgnd/Virtual Sensors/Battery/BattRes ==
  note: TBC
  Data : Inport
  Bus Selector : BusSelector  Commented=on  OutputSignals=VirtualSensors.Batt.BattRes [ohm]
  Bus Selector1 : BusSelector  OutputSignals=Sensors.CAN.Batt.BMS2_VoltageSOC.Batt_SOC.Batt_SOC [],VirtualSensors.Batt.BattCellTempAvg [degC]
  Ground : Ground
  Header : Blocks_lib/Header  width=Portrait  addtext=''
  Multiport Switch : MultiPortSwitch  DataPortOrder=Zero-based contiguous  Inputs=2  zeroidx=on
  raptor_adjustment : Raptor_lib/Data Storage/raptor_adjustment  paramName='BattResOption'  nameSource=Parameter  initValue=0  dataType=uint8  storage=Calibration  calDispType=Enumeration  calEnum={'BMS', 'Model'}  calGain=1  calOffset=0  calMax=inf  calMin=-inf  calFormat=''  calUnit=''  calHelp='Battery resistance option'  calAccess=1  calFunction='Virtual Sensors | Battery'  calDispHeaders=off  calColHeaders={'Col1' 'Col2' 'Col3'}  calRowHeaders={'Row1' 'Row2' 'Row3'}
      settings: SourceProductName=Raptor
  raptor_measurement : Raptor_lib/Data Storage/raptor_measurement  paramName='BattResFinal'  nameSource=Parameter  calDispType=Number  calEnum={'Disabled', 'Enabled'}  calGain=1  calOffset=0  calMax=inf  calMin=-inf  calFormat=''  calUnit='ohm'  calHelp='Battery resistance'  calAccess=1  calFunction='Virtual Sensors | Battery'  calVisible=on
      settings: SourceProductName=Raptor
  raptor_table_2d : Raptor_lib/Table Lookup/raptor_table_2d  dataName='BattResMap'  initValue=zeros(11,11)  dataType=double  storage=Calibration  initValueX=[1:11]  initValueY=[1:11]  dataTypeXY=double  storageXY=Calibration  calVisible=on  showTable=on  calGain=1.0  calOffset=0.0  calMax=Inf  calMin=-Inf  calFormat='-1'  calUnit='ohm'  calHelp='Battery resistance'  showBreakpointX=on  dataNameX='BattCellTempAvg11IdxArr'  calGainX=1.0  calOffsetX=0.0  calMaxX=Inf  calMinX=-Inf  calFormatX='-1'  calUnitX='degC'  calHelpX='Index array'  showBreakpointY=on  dataNameY='BattSOC11IdxArr'  calGainY=1.0  calOffsetY=0.0  calMaxY=Inf  calMinY=-Inf  calFormatY='-1'  calUnitY='%'  calHelpY='Index array'  calAccess=1  calFunction='Virtual Sensors | Battery'  measureEnable=on  mName='BattResMap_out'
      settings: SourceProductName=Raptor
  ohm : Outport  VectorParamsAs1DForOutWhenUnconnected=off
  wires:
  raptor_adjustment/1 -> Multiport Switch/1
  raptor_table_2d/1 -> Multiport Switch/3
  Multiport Switch/1 -> raptor_measurement/1, ohm/1
  Bus Selector1/2 -> raptor_table_2d/2  "<BattCellTempAvg [degC]>"
  Bus Selector1/1 -> raptor_table_2d/1  "<Batt_SOC []>"
  Data/1 -> Bus Selector/1, Bus Selector1/1
  Ground/1 -> Multiport Switch/2

== system VCMGCM1962020b_v2/Fgnd/Virtual Sensors/Battery/BattVoltOC ==
  note: TBC
  Data : Inport
  Bus Selector : BusSelector  OutputSignals=VirtualSensors.Batt.BattRes [ohm]
  Constant : Constant  Value=0
  Fcn : Fcn  Expr=u(1) + u(2) * u(3)
  First-Order Filter : Blocks_lib/Filt  nam='BattVoltOCFiltTC'  group='Virtual Sensors | Battery'  samptime=samptime
  Header : Blocks_lib/Header  width=Portrait  addtext=''
  Mux : Mux  Inputs=3
  raptor_measurement : Raptor_lib/Data Storage/raptor_measurement  paramName='BattVoltOC'  nameSource=Parameter  calDispType=Number  calEnum={'Disabled', 'Enabled'}  calGain=1  calOffset=0  calMax=inf  calMin=-inf  calFormat=''  calUnit='V'  calHelp='Battery pack voltage (open-circuit)'  calAccess=1  calFunction='Virtual Sensors | Battery'  calVisible=on
      settings: SourceProductName=Raptor
  V : Outport  VectorParamsAs1DForOutWhenUnconnected=off
  wires:
  First-Order Filter/1 -> V/1, raptor_measurement/1
  Fcn/1 -> First-Order Filter/1
  Mux/1 -> Fcn/1
  Data/1 -> Bus Selector/1
  Bus Selector/1 -> Mux/1  "<BattRes [ohm]>"
  Constant/1 -> Mux/3
  ? -> Mux/2  "<Batt_Current []>"

== system VCMGCM1962020b_v2/Fgnd/Virtual Sensors/Charger/ChgPlugState ==
  note: TBC
  Data : Inport
  AND : Logic  AllPortsSameDT=off  OutDataTypeStr=boolean
  Bus Selector : BusSelector  OutputSignals=Sensors.Sensors.Volt.WakeChgr.WakeChgrVld [Bool],Sensors.Sensors.Volt.WakeChgr.WakeChgr [Bool]
  CmprTo : Blocks_lib/CmprTo  op===  val='Connected'  enum=EnumLst.ChgPlugState
  EnumCnst : Blocks_lib/EnumCnst  val='Disconnected'  typ=uint8  enum=EnumLst.ChgPlugState
  EnumCnst1 : Blocks_lib/EnumCnst  val='Connected'  typ=uint8  enum=EnumLst.ChgPlugState
  Header : Blocks_lib/Header  width=Portrait  addtext=''
  Multiport Switch : MultiPortSwitch  DataPortOrder=Zero-based contiguous  Inputs=2  DataPortIndices={0, 6, 7}  zeroidx=on
  enum : Outport  VectorParamsAs1DForOutWhenUnconnected=off
  wires:
  Data/1 -> Bus Selector/1
  EnumCnst/1 -> Multiport Switch/2
  EnumCnst1/1 -> Multiport Switch/3
  CmprTo/1 -> enum/1
  Bus Selector/1 -> AND/1  "<WakeChgrVld [Bool]>"
  Bus Selector/2 -> AND/2  "<WakeChgr [Bool]>"
  AND/1 -> Multiport Switch/1
  Multiport Switch/1 -> CmprTo/1

== system VCMGCM1962020b_v2/Fgnd/Virtual Sensors/Charger/ChgPortDCVolt ==
  Data : Inport
  Bus Selector : BusSelector  OutputSignals=Sensors.CAN.Other.ChgPortDCVolt.cs_ivt_msg_result_voltage_ch1.result_volt_ch1_meas_value.result_volt_ch1_meas_valueVld [Bool],Sensors.CAN.Other.ChgPortDCVolt.cs_ivt_msg_result_voltage_ch1.result_volt_ch1_meas_value.result_volt_ch1_meas_value []
  Header : Blocks_lib/Header  width=Portrait  addtext=''
  Zero-Order Hold : ZeroOrderHold  SampleTime=-1
  mV to V : Gain  Gain=0.001
  Vld : Outport  VectorParamsAs1DForOutWhenUnconnected=off
  V : Outport  Port=2  VectorParamsAs1DForOutWhenUnconnected=off
  wires:
  mV to V/1 -> V/1
  Data/1 -> Bus Selector/1
  Bus Selector/2 -> mV to V/1  "<result_volt_ch1_meas_value []>"
  Zero-Order Hold/1 -> Vld/1
  Bus Selector/1 -> Zero-Order Hold/1  "<result_volt_ch1_meas_valueVld [Bool]>"

== system VCMGCM1962020b_v2/Fgnd/Virtual Sensors/Charger/Off Board ==
  Data : Inport
  Bus Creator : BusCreator  Inputs=9
  Bus Selector : BusSelector  OutputSignals=Actuators.CAN.CCS.Cmd.BattIsoTestDsbl [Bool],Actuators.CAN.CCS.Cmd.DCChgCntr [Bool]
  Bus Selector1 : BusSelector  OutputSignals=Sensors.CAN.CCS.CCSEVSE_DC_ChargeInfo1.CCSEVSEPresentCurrent.CCSEVSEPresentCurrentVld [Bool],Sensors.CAN.CCS.CCSEVSE_DC_ChargeInfo1.CCSEVSEPresentCurrent.CCSEVSEPresentCurrent [A],Sensors.CAN.CCS.CCSEVSE_ChargeParameters1.CCSEVSEMaximumCurrentLimit.CCSEVSEMaximumCurrentLimit [A]
  Header : Blocks_lib/Header  width=Portrait  addtext=''
  OffBoardChgr : Subsystem
  OffBoardChgrIsoFault : Subsystem
  OffBoardChgrShutdown : Subsystem
  Zero-Order Hold{,1..4} (5 alike) : ZeroOrderHold  SampleTime=-1
  " Data" : Outport  VectorParamsAs1DForOutWhenUnconnected=off
  wires:
  Bus Creator/1 -> " Data"/1  "OffBoard"
  OffBoardChgr/1(Bool) -> Bus Creator/1  "OffBoardChgr [Bool]"
  Data/1 -> OffBoardChgr/1(Data), Bus Selector/1, Bus Selector1/1, OffBoardChgrShutdown/1(Data), OffBoardChgrIsoFault/1(Data)
  OffBoardChgrShutdown/1(Bool) -> Bus Creator/6  "OffBoardChgrShutdown [Bool]"
  Zero-Order Hold2/1 -> Bus Creator/8  "OffBoardChgrDCCur [A]"
  Bus Selector/1 -> Zero-Order Hold/1  "<BattIsoTestDsbl [Bool]>"
  Zero-Order Hold/1 -> Bus Creator/4  "OffBoardChgrHVBusIsoTestDsbl [Bool]"
  Bus Selector1/2 -> Zero-Order Hold2/1  "<CCSEVSEPresentCurrent [A]>"
  Bus Selector1/3 -> Zero-Order Hold3/1  "<CCSEVSEMaximumCurrentLimit [A]>"
  Zero-Order Hold3/1 -> Bus Creator/9  "OffBoardChgrEVSEDCCurLim [A]"
  Zero-Order Hold1/1 -> Bus Creator/7  "OffBoardChgrDCCurVld [Bool]"
  OffBoardChgrIsoFault/1(Vld) -> Bus Creator/2  "OffBoardChgrIsoFaultVld [Bool]"
  Bus Selector1/1 -> Zero-Order Hold1/1  "<CCSEVSEPresentCurrentVld [Bool]>"
  Zero-Order Hold4/1 -> Bus Creator/5  "OffBoardChgrDCChgCntrReq [Bool]"
  Bus Selector/2 -> Zero-Order Hold4/1  "<DCChgCntr [Bool]>"
  OffBoardChgrIsoFault/2(Bool) -> Bus Creator/3  "OffBoardChgrIsoFault [Bool]"

== system VCMGCM1962020b_v2/Fgnd/Virtual Sensors/Charger/On Board ==
  note: TBC
  Data : Inport
  Bus Creator : BusCreator  Inputs=10
  Bus Selector : BusSelector  OutputSignals=Sensors.CAN.OnBoardChgr.ChgrCCSA.ChgrChrgr_Out_curr.ChgrChrgr_Out_currVld [Bool],Sensors.CAN.OnBoardChgr.ChgrCCSA.ChgrChrgr_Out_curr.ChgrChrgr_Out_curr [A]
  Bus Selector1 : BusSelector  OutputSignals=Sensors.CAN.OnBoardChgr.ChgrCCSA.ChgrChrgr_Out_volt.ChgrChrgr_Out_volt [V],Sensors.CAN.OnBoardChgr.ChgrCCSA.ChgrChrgr_internal_temp.ChgrChrgr_internal_temp [C],Sensors.CAN.OnBoardChgr.ChgrCCSA.ChgrChargr_temp_flag.ChgrChargr_temp_flag [enum]
  Constant1 : Constant  Value=false
  Header : Blocks_lib/Header  width=Portrait  addtext=''
  OnBoardChgr : Subsystem
  OnBoardChgrFault : Subsystem
  Zero-Order Hold{,1..5,7} (7 alike) : ZeroOrderHold  SampleTime=-1
  raptor_adjustment : Raptor_lib/Data Storage/raptor_adjustment  paramName='OBC_EVSE_CurrLim'  nameSource=Parameter  initValue=10  dataType=double  storage=Calibration  calDispType=Number  calEnum={'False', 'True'}  calGain=1.0  calOffset=0.0  calMax=inf  calMin=-inf  calFormat='-1'  calUnit='A'  calHelp='Current limit for EVSE '  calAccess=1  calFunction='Virtual Sensor | Charger'  calDispHeaders=off  calColHeaders={'Col1' 'Col2' 'Col3'}  calRowHeaders={'Row1' 'Row2' 'Row3'}
      settings: SourceProductName=Raptor
  " Data" : Outport  VectorParamsAs1DForOutWhenUnconnected=off
  wires:
  Bus Creator/1 -> " Data"/1
  OnBoardChgr/1(Bool) -> Bus Creator/1  "OnBoardChgr [Bool]"
  Zero-Order Hold3/1 -> Bus Creator/7  "OnBoardChgrTemp [degC]"
  Data/1 -> OnBoardChgr/1(Data), Bus Selector/1, Bus Selector1/1, OnBoardChgrFault/1(Data)
  Zero-Order Hold2/1 -> Bus Creator/6  "OnBoardChgrDCVolt [V]"
  Zero-Order Hold/1 -> Bus Creator/4  "OnBoardChgrEVSEACCurLim [A]"
  Zero-Order Hold1/1 -> Bus Creator/5  "OnBoardChgrDCVoltVld [Bool]"
  OnBoardChgrFault/1(Vld) -> Bus Creator/2  "OnBoardChgrFaultVld [Bool]"
  OnBoardChgrFault/2(Bool) -> Bus Creator/3  "OnBoardChgrFault [Bool]"
  Constant1/1 -> Zero-Order Hold1/1
  raptor_adjustment/1 -> Zero-Order Hold/1
  Bus Selector/2 -> Zero-Order Hold5/1  "<ChgrChrgr_Out_curr [A]>"
  Bus Selector/1 -> Zero-Order Hold4/1  "<ChgrChrgr_Out_currVld [Bool]>"
  Zero-Order Hold4/1 -> Bus Creator/9  "OnBoardChgCurVld [Bool]"
  Zero-Order Hold5/1 -> Bus Creator/10  "OnBoardChgrOutCur [A]"
  Bus Selector1/2 -> Zero-Order Hold3/1  "<ChgrChrgr_internal_temp [C]>"
  Bus Selector1/1 -> Zero-Order Hold2/1  "<ChgrChrgr_Out_volt [V]>"
  Bus Selector1/3 -> Zero-Order Hold7/1  "<ChgrChargr_temp_flag [enum]>"
  Zero-Order Hold7/1 -> Bus Creator/8  "OnBoardChgrOverTemp [Bool]"

== system VCMGCM1962020b_v2/Fgnd/Virtual Sensors/DC//DC Converter/DCDCFault ==
  Data : Inport
  Bus Selector1 : BusSelector  OutputSignals=Sensors.CAN.DCDC.DCDC_Status_0_16V.DCDC_Status_0_16VMsgVld [Bool],Sensors.CAN.DCDC.DCDC_Status_0_16V.Fault_alarm1_0_16V.Fault_alarm1_0_16V []
  Compare To Constant : simulink/Logic and Bit Operations/Compare To Constant  relop=~=  const=0  OutDataTypeStr=boolean
  Header : Blocks_lib/Header  width=Portrait  addtext=''
  Vld : Outport  VectorParamsAs1DForOutWhenUnconnected=off
  Bool : Outport  Port=2  VectorParamsAs1DForOutWhenUnconnected=off
  wires:
  Compare To Constant/1 -> Bool/1
  Data/1 -> Bus Selector1/1
  Bus Selector1/1 -> Vld/1  "<DCDC_Status_0_16VMsgVld [Bool]>"
  Bus Selector1/2 -> Compare To Constant/1  "<Fault_alarm1_0_16V []>"

== system VCMGCM1962020b_v2/Fgnd/Virtual Sensors/DC//DC Converter/DCDCInptCur ==
  Data : Inport
  Bus Selector : BusSelector  OutputSignals=Sensors.CAN.DCDC.DCDC_Status_0_16V.DCDCOutput_Voltage_0_16V.DCDCOutput_Voltage_0_16V [V],Sensors.CAN.DCDC.DCDC_Status_0_16V.DCDC_Output_Current_0_16V.DCDC_Output_Current_0_16V [A],VirtualSensors.PDU.HVBusVolt [V]
  Eqn(w/DvdByZeroPro) : Blocks_lib/Eqn(w//DvdByZeroPro)  eqn='u(1) * u(2) / (u(3) * u(4) / 100)'  dmn='(u(3) * u(4) / 100)'  dfltval=0
  Header : Blocks_lib/Header  width=Portrait  addtext=''
  Mux : Mux
  raptor_adjustment : Raptor_lib/Data Storage/raptor_adjustment  paramName='DCDCEff'  nameSource=Parameter  initValue=0  dataType=double  storage=Calibration  calDispType=Number  calEnum={'Disabled', 'Enabled'}  calGain=1  calOffset=0  calMax=inf  calMin=-inf  calFormat=''  calUnit='%'  calHelp='DC/DC converter efficiency'  calAccess=1  calFunction='Virtual Sensors | PDU'  calDispHeaders=off  calColHeaders={'Col1' 'Col2' 'Col3'}  calRowHeaders={'Row1' 'Row2' 'Row3'}
      settings: SourceProductName=Raptor
  raptor_measurement : Raptor_lib/Data Storage/raptor_measurement  paramName='DCDCInptCur'  nameSource=Parameter  calDispType=Number  calEnum={'Disabled', 'Enabled'}  calGain=1  calOffset=0  calMax=inf  calMin=-inf  calFormat=''  calUnit='A'  calHelp='DC/DC converter input current'  calAccess=1  calFunction='Virtual Sensors | PDU'  calVisible=on
      settings: SourceProductName=Raptor
  A : Outport  VectorParamsAs1DForOutWhenUnconnected=off
  wires:
  Mux/1 -> Eqn(w/DvdByZeroPro)/1
  Bus Selector/3 -> Mux/3  "<HVBusVolt [V]>"
  Bus Selector/2 -> Mux/2  "<DCDC_Output_Current_0_16V [A]>"
  Bus Selector/1 -> Mux/1  "<DCDCOutput_Voltage_0_16V [V]>"
  raptor_adjustment/1 -> Mux/4
  Eqn(w/DvdByZeroPro)/1 -> A/1, raptor_measurement/1
  Data/1 -> Bus Selector/1

== system VCMGCM1962020b_v2/Fgnd/Virtual Sensors/Drive Inverter/DrvInvtrCur ==
  Data : Inport
  Bus Selector1 : BusSelector  OutputSignals=Sensors.CAN.DrvInvtr.EM3.EM3PhCur.EM3_PhaseAmpsRms.EM3_PhaseAmpsRmsVld [Bool],Sensors.CAN.DrvInvtr.EM3.EM3PhCur.EM3_PhaseAmpsRms.EM3_PhaseAmpsRms [A]
  Header : Blocks_lib/Header  width=Portrait  addtext=''
  Product : Product
  Zero-Order Hold : ZeroOrderHold  SampleTime=-1
  raptor_adjustment : Raptor_lib/Data Storage/raptor_adjustment  paramName='DataName'  nameSource=Parameter  initValue=1.35  dataType=double  storage=Calibration  calDispType=Number  calEnum={'False', 'True'}  calGain=1.0  calOffset=0.0  calMax=inf  calMin=-inf  calFormat='-1'  calUnit='nd'  calHelp='3phase rms to DC factor'  calAccess=1  calFunction='Virtual Sensors | Invtr'  calDispHeaders=off  calColHeaders={'Col1' 'Col2' 'Col3'}  calRowHeaders={'Row1' 'Row2' 'Row3'}
      settings: SourceProductName=Raptor
  Vld : Outport  VectorParamsAs1DForOutWhenUnconnected=off
  A : Outport  Port=2  VectorParamsAs1DForOutWhenUnconnected=off
  wires:
  Bus Selector1/1 -> Zero-Order Hold/1  "<EM3_PhaseAmpsRmsVld [Bool]>"
  Data/1 -> Bus Selector1/1
  Product/1 -> A/1
  raptor_adjustment/1 -> Product/2
  Zero-Order Hold/1 -> Vld/1
  Bus Selector1/2 -> Product/1  "<EM3_PhaseAmpsRms [A]>"

== system VCMGCM1962020b_v2/Fgnd/Virtual Sensors/Drive Inverter/DrvInvtrFault ==
  Data : Inport
  Bus Selector : BusSelector  OutputSignals=Sensors.CAN.DrvInvtr.EM1.EM1MsgVld [Bool],Sensors.CAN.DrvInvtr.EM1.EM1_eIgbtPhCErr.EM1_eIgbtPhCErr [],Sensors.CAN.DrvInvtr.EM1.EM1_eIgbtPhBErr.EM1_eIgbtPhBErr [],Sensors.CAN.DrvInvtr.EM1.EM1_eIgbtPhAErr.EM1_eIgbtPhAErr [],Sensors.CAN.DrvInvtr.EM1.EM1_eGeneric.EM1_eGeneric [],Sensors.CAN.DrvInvtr.EM1.EM1_eSysInit.EM1_eSysInit [],Sensors.CAN.DrvInvtr.EM1.EM1_eLogicSuppFault.EM1_eLogicSuppFault [],Sensors.CAN.DrvInvtr.EM1.EM1_eBridgeFault.EM1_eBridgeFault []
  Header : Blocks_lib/Header  width=Portrait  addtext=''
  Logical Operator : Logic  Operator=OR  Inputs=1  OutDataTypeStr=boolean
  Mux : Mux  Inputs=7
  Zero-Order Hold : ZeroOrderHold  SampleTime=-1
  Vld : Outport  VectorParamsAs1DForOutWhenUnconnected=off
  Bool : Outport  Port=2  VectorParamsAs1DForOutWhenUnconnected=off
  wires:
  Logical Operator/1 -> Bool/1
  Mux/1 -> Logical Operator/1
  Data/1 -> Bus Selector/1
  Bus Selector/2 -> Mux/1  "<EM1_eIgbtPhCErr []>"
  Zero-Order Hold/1 -> Vld/1
  Bus Selector/1 -> Zero-Order Hold/1  "<EM1MsgVld [Bool]>"
  Bus Selector/3 -> Mux/2  "<EM1_eIgbtPhBErr []>"
  Bus Selector/4 -> Mux/3  "<EM1_eIgbtPhAErr []>"
  Bus Selector/5 -> Mux/4  "<EM1_eGeneric []>"
  Bus Selector/6 -> Mux/5  "<EM1_eSysInit []>"
  Bus Selector/7 -> Mux/6  "<EM1_eLogicSuppFault []>"
  Bus Selector/8 -> Mux/7  "<EM1_eBridgeFault []>"

== system VCMGCM1962020b_v2/Fgnd/Virtual Sensors/Drive Inverter/DrvMtrTmp ==
  Data : Inport
  Bus Selector : BusSelector  OutputSignals=Sensors.CAN.DrvInvtr.EM2.EM2MtrTemp.EM2_MotorSensorTemp.EM2_MotorSensorTemp [degC]
  Header : Blocks_lib/Header  width=Portrait  addtext=''
  Zero-Order Hold : ZeroOrderHold  SampleTime=-1
  degC : Outport  VectorParamsAs1DForOutWhenUnconnected=off
  wires:
  Data/1 -> Bus Selector/1
  Bus Selector/1 -> Zero-Order Hold/1  "<EM2_MotorSensorTemp [degC]>"
  Zero-Order Hold/1 -> degC/1

== system VCMGCM1962020b_v2/Fgnd/Virtual Sensors/Driver Inputs/APP ==
  Data : Inport
  Arb : Blocks_lib/Arb  nam='APP'  units='%'  eqn='(u(1) + u(2)) / 2'  minmax=min  samptime=samptime
  Bus Selector : BusSelector  OutputSignals=Sensors.Sensors.Driver.APP1.APP1Vld [Bool],Sensors.Sensors.Driver.APP2.APP2Vld [Bool],Sensors.Sensors.Driver.APP1.APP1 [%],Sensors.Sensors.Driver.APP2.APP2 [%]
  Bus Selector2 : BusSelector  OutputSignals=Sensors.Sensors.Driver.APP1.APP1Vld [Bool],Sensors.Sensors.Driver.APP1ADC [ADC]
  Bus Selector3 : BusSelector  OutputSignals=Sensors.Sensors.Driver.APP2.APP2Vld [Bool],Sensors.Sensors.Driver.APP2ADC [ADC]
  Ddbnd(PctInpt) : Blocks_lib/Ddbnd(PctInpt)  nam='APP'  group='Virtual Sensors | Driver Input'
  Header : Blocks_lib/Header  width=Portrait  addtext=''
  Learn-Up Enable : Subsystem
  Meas&Ovrd : Blocks_lib/Meas&Ovrd  nam='APP'  name_source=Parameter  view_as=Number  enum_struct={}  gain=1  min=-inf  max=inf  precision=''  units='%'  help='Accelerator pedal position'  group='Virtual Sensors | Driver Input'
  SnsLinPctAdapt : Blocks_lib/SnsLinPctAdapt  nam='APP1'  group='Virtual Sensors | Driver Input'  samptime=samptime
  SnsLinPctAdapt1 : Blocks_lib/SnsLinPctAdapt  nam='APP2'  group='Virtual Sensors | Driver Input'  samptime=samptime
  Vld : Outport  VectorParamsAs1DForOutWhenUnconnected=off
  % : Outport  Port=2  VectorParamsAs1DForOutWhenUnconnected=off
  wires:
  Data/1 -> Bus Selector3/1, Learn-Up Enable/1(Data), Bus Selector2/1, Bus Selector/1
  Arb/1 -> Vld/1
  Meas&Ovrd/1 -> %/1
  Bus Selector3/2 -> SnsLinPctAdapt1/2  "<APP2ADC [ADC]>"
  Bus Selector3/1 -> SnsLinPctAdapt1/1  "<APP2Vld [Bool]>"
  Learn-Up Enable/1(Bool) -> SnsLinPctAdapt1/3, SnsLinPctAdapt/3
  Bus Selector2/2 -> SnsLinPctAdapt/2  "<APP1ADC [ADC]>"
  Bus Selector2/1 -> SnsLinPctAdapt/1  "<APP1Vld [Bool]>"
  Bus Selector/4 -> Arb/4  "<APP2 [%]>"
  Bus Selector/3 -> Arb/3  "<APP1 [%]>"
  Bus Selector/2 -> Arb/2  "<APP2Vld [Bool]>"
  Bus Selector/1 -> Arb/1  "<APP1Vld [Bool]>"
  Arb/2 -> Ddbnd(PctInpt)/1
  Ddbnd(PctInpt)/1 -> Meas&Ovrd/1
